simulink model "PID_analytic"  (R2019a)
settings: Solver=ode4  StartTime=0.0  StopTime=100  FixedStep=0.01  RelTol=1e-3
values from neighbouring files (symbols this model uses):
  operPoint = [x0(i); y0(i); z0(i)]    [Control.m]
  q0 = double(solutions.q0s)    [Control.m]
  q1 = double(solutions.q1s)    [Control.m]
  q2 = double(solutions.q2s)    [Control.m]
  r1 = double(solutions.r1s)    [Control.m]
  systemD = c2d(system,1)    [Control.m]
  T = 1    [Control.m]
settings Model: Creator=Mateo  LastModifiedBy=Juan
settings DataIOCC: SaveFormat=Array  SignalLogging=off  DSMLogging=off  ReturnWorkspaceOutputs=off

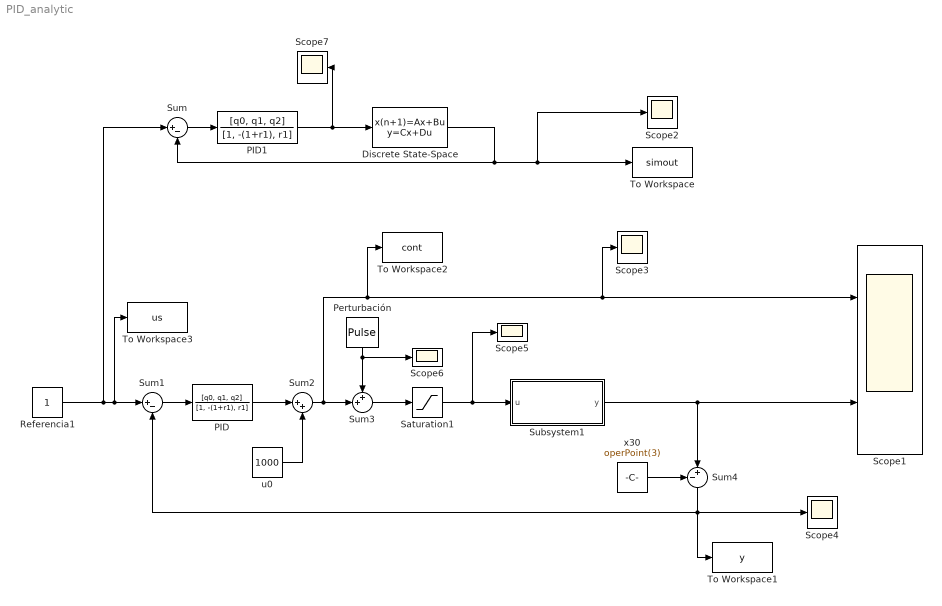
== system PID_analytic ==
  " Perturbación" : DiscretePulseGenerator  PulseType=Time based  Amplitude=0  Period=10  PulseWidth=5
  Discrete State-Space : DiscreteStateSpace  A=systemD.A  B=systemD.B  C=systemD.C  D=systemD.D  InitialCondition=[0,0,0]
  PID : DiscreteTransferFcn  Numerator=[q0, q1, q2]  Denominator=[1, -(1+r1), r1]  SampleTime=T
  PID1 : DiscreteTransferFcn  Numerator=[q0, q1, q2]  Denominator=[1, -(1+r1), r1]  SampleTime=T
  Referencia1 : Constant
  Saturation1 : Saturate  UpperLimit=1500  LowerLimit=0
  Scope1 : Scope  NumInputPorts=2
  Scope{2..7} (6 alike) : Scope
  Subsystem1 : Subsystem  mask{Ra=300, Rb=7500, Rc=17.5439, RCs=1, ci=operPoint}
      mask prompts: Ra "Resistance a"; Rb "Resistance b"; Rc "Resistance c"; RCs "Time speed (RC)"; ci "Initial Conditions"
      mask init:
      | x10 = ci(1);
      | x20 = ci(2);
      | y0 = ci(3);
      mask Display: disp("Rössler Attractor")
  Sum : Sum  Inputs=|+-
  Sum1 : Sum  Inputs=|+-
  Sum2 : Sum  Inputs=|++
  Sum3 : Sum  Inputs=++|
  Sum4 : Sum  Inputs=-+|
  To Workspace : ToWorkspace  VariableName=simout  SampleTime=-1
  To Workspace1 : ToWorkspace  VariableName=y  SampleTime=-1
  To Workspace2 : ToWorkspace  VariableName=cont  SampleTime=0.01
  To Workspace3 : ToWorkspace  VariableName=us  SampleTime=-1
  u0 : Constant  Value=1000
  x30 : Constant  Value=operPoint(3)
  wires:
  PID1/1 -> Discrete State-Space/1, Scope7/1
  Saturation1/1 -> Subsystem1/1(u), Scope5/1
  Discrete State-Space/1 -> Sum/2, Scope2/1, To Workspace/1
  Sum2/1 -> Sum3/2, To Workspace2/1, Scope3/1, Scope1/1
  Sum1/1 -> PID/1
  " Perturbación"/1 -> Sum3/1, Scope6/1
  Sum4/1 -> To Workspace1/1, Scope4/1, Sum1/2
  Referencia1/1 -> Sum/1, To Workspace3/1, Sum1/1
  x30/1 -> Sum4/1
  PID/1 -> Sum2/1
  Sum3/1 -> Saturation1/1
  Sum/1 -> PID1/1
  u0/1 -> Sum2/2
  Subsystem1/1("y ") -> Scope1/2, Sum4/2

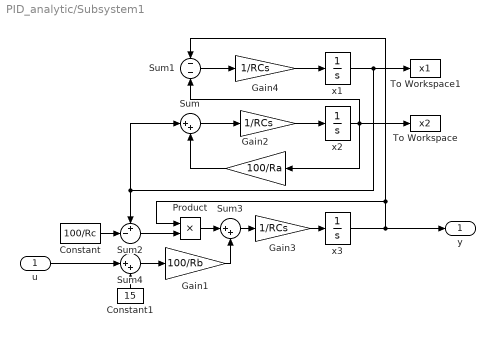
== system PID_analytic/Subsystem1 ==
  u : Inport
  " " : Gain  Gain=1/RCs
  Constant : Constant  Value=100/Rc
  Constant1 : Constant  Value=15
  Gain1 : Gain  Gain=100/Rb
  Gain2 : Gain  Gain=100/Ra
  Gain3 : Gain  Gain=1/RCs
  Gain4 : Gain  Gain=1/RCs
  Product : Product
  Sum : Sum  Inputs=|++
  Sum1 : Sum  Inputs=--
  Sum2 : Sum  Inputs=+-|
  Sum3 : Sum  Inputs=|++
  Sum4 : Sum  Inputs=|++
  To Workspace : ToWorkspace  VariableName=x2  SampleTime=-1
  To Workspace1 : ToWorkspace  VariableName=x1  SampleTime=-1
  x1 : Integrator  InitialCondition=x10
  x2 : Integrator  InitialCondition=x20
  "x3 " : Integrator  InitialCondition=y0
  "y " : Outport
  wires:
  Sum1/1 -> Gain4/1
  Gain2/1 -> Sum/2
  Sum2/1 -> Product/2
  Product/1 -> Sum3/1
  "x3 "/1 -> "y "/1, Sum1/1, Product/1
  x1/1 -> To Workspace1/1, Sum2/1, Sum/1
  Sum/1 -> " "/1
  Sum3/1 -> Gain3/1
  Constant/1 -> Sum2/2
  x2/1 -> Sum1/2, To Workspace/1, Gain2/1
  u/1 -> Sum4/1
  " "/1 -> x2/1
  Gain3/1 -> "x3 "/1
  Gain4/1 -> x1/1
  Gain1/1 -> Sum3/2
  Constant1/1 -> Sum4/2
  Sum4/1 -> Gain1/1
